simulink model "Collision_05_Disk_in_Ring"  (R2014a)
settings: Solver=ode15s  StartTime=0.0  StopTime=5  MaxStep=1e-2  RelTol=1e-4  AbsTol=1e-5
PostLoadFcn:
  | warning off Simulink:Engine:UsingDefaultMaxStepSize
StartFcn:
  | tic;
StopFcn:
  | Elapsed_Sim_Time = toc;
  | disp(['Elapsed Sim Time = ' num2str(Elapsed_Sim_Time)]);
undefined symbols (not defined in the file): X, Y, Z
libraries: sm_lib x6, Parts_Lib x2, nesl_utility x2, Contact_Forces_Lib x1
Description:
  | Copyright 2014 The MathWorks, Inc.
settings Model: Creator=smiller  LastModifiedBy=smiller
settings SolverCC: ZeroCrossAlgorithm=Adaptive
settings DataIOCC: LimitDataPoints=off
settings OptimizationCC: ExpressionDepthLimit=2147483647
settings DebuggingCC: UnderspecifiedInitializationDetection=Classic  IgnoredZcDiagnostic=none  FcnCallInpInsideContextMsg=EnableAllAsWarning  StateNameClashWarn=warning
settings DiagnosticsConfigSet: SimMechanicsRigidlyBoundBlock=none
settings ExplorerConfigSet: InternalSimMechanicsExplorerSettings="<ExplorerConfiguration><canonicalview>default</canonicalview><AnimationSetting><BasePlaybackSpeed>1.0</BasePlaybackSpeed><PlaybackSpeedFactor>1.0</PlaybackSpeedFactor></AnimationSetting><TilePanel><TileInfo><Tiles Columns=\"1\" Count=\"1\" Rows=\"1\"><Column Left=\"2\" Weight=\"1\"/><Column Left=\"392\"/><Row Top=\"2\" Weight=\"1\"/><Row Top=\"346\"/><Tile Height=\"1\" Width=\"1\" X=\"0\" Y=\"0\"/></Tiles></TileInfo><SceneInfo><SceneViewer><BGColor><R>0.92549020051956177</R><G>0.94901961088180542</G><B>0.94901961088180542</B></BGColor><Camera><Position><X>0.30265771427387711</X><Y>-0.55071230602769961</Y><Z>0.10379549062534259</Z></Position><Center><X>0.0025347841246010638</X><Y>0.0091500402941713244</Y><Z>0.0013498174437712174</Z></Center><Up><X>-0.17021912957199431</X><Y>0.088338633384022841</Y><Z>0.98143860418244988</Z></Up><Left>-0.23099999874830246</Left><Right>0.23099999874830246</Right><Bottom>-0.23099999874830246</Bottom><Top>0.23099999874830246</Top></Camera></SceneViewer></SceneInfo></TilePanel></ExplorerConfiguration>"

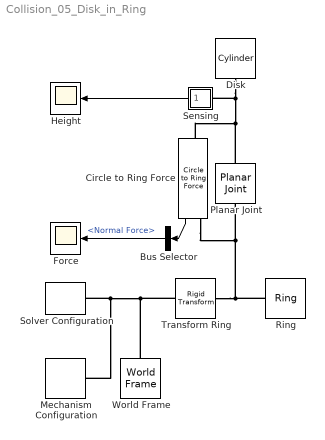
== system Collision_05_Disk_in_Ring ==
  Bus Selector : BusSelector  OutputSignals=Normal Force
  Circle to Ring Force : Contact_Forces_Lib/2D/Circle to Ring Force  radius_circle=0.05  radius_ring=0.21  d_ring=0.02  active_angle=[-180 180]  force_law=Linear  k_contact=1e4  b_contact=1e1  pen_full_damp_F=1e-4  pen_exponent=1  custom_param_1=1  custom_param_2=1  friction_law=None  mu_kinetic=0.5  mu_static=0.7  v_thr=0.001
  Disk : Parts_Lib/Cylinder  cyl_radius=0.05  cyl_length=0.05  cyl_density=1000  cyl_color=red  mark_radius=[0.75 0.5]  mark_angle=60  mark_color=purple
  Force : Scope
      settings: TimeRange=5  YMin=0  YMax=150
  Height : Scope
      settings: YMin=-0.2  YMax=0.2
  Mechanism Configuration : sm_lib/Utilities/Mechanism Configuration  UniformGravity=Constant  GravityVector=[0 0 -9.81]  GravityUnits=m/s^2  LinearizationDelta=0.001  BlockFunction=simmechanics.library.utilities.mechanism_configuration
  Planar Joint : sm_lib/Joints/Planar Joint  SenseConstraintForce=off  SenseConstraintForceX=off  SenseConstraintForceY=off  SenseConstraintForceZ=off  SenseConstraintTorque=off  SenseConstraintTorqueX=off  SenseConstraintTorqueY=off  SenseConstraintTorqueZ=off  SenseTotalForce=off  SenseTotalForceX=off  SenseTotalForceY=off  SenseTotalForceZ=off  SenseTotalTorque=off  SenseTotalTorqueX=off  SenseTotalTorqueY=off  SenseTotalTorqueZ=off  CompositeWrenchDir=FollowerOnBase  CompositeWrenchFrame=BaseFrame  PxEquilibriumPosition=0  PxEquilibriumPositionUnits=m  PxSpringStiffness=0  PxSpringStiffnessUnits=N/m  PxDampingCoefficient=0  PxDampingCoefficientUnits=N/(m/s)  PxTorqueActuationMode=NoTorque  PxMotionActuationMode=ComputedMotion  PxSensePosition=off  PxSenseVelocity=off  PxSenseAcceleration=off  PxSenseTorqueForce=off  PxPositionTargetValue=0.07  PxPositionTargetValueUnits=m  PxPositionTargetSpecify=on  PxPositionTargetPriority=High  PxVelocityTargetValue=0  PxVelocityTargetValueUnits=m/s  PxVelocityTargetSpecify=off  PxVelocityTargetPriority=High  PyEquilibriumPosition=0  PyEquilibriumPositionUnits=m  PySpringStiffness=0  PySpringStiffnessUnits=N/m  PyDampingCoefficient=0  PyDampingCoefficientUnits=N/(m/s)  PyTorqueActuationMode=NoTorque  PyMotionActuationMode=ComputedMotion  PySensePosition=off  PySenseVelocity=off  PySenseAcceleration=off  PySenseTorqueForce=off  PyPositionTargetValue=0.05  PyPositionTargetValueUnits=m  PyPositionTargetSpecify=on  PyPositionTargetPriority=High  PyVelocityTargetValue=0.5*0  PyVelocityTargetValueUnits=m/s  PyVelocityTargetSpecify=on  PyVelocityTargetPriority=High  RzEquilibriumPosition=0  RzEquilibriumPositionUnits=deg  RzSpringStiffness=0  RzSpringStiffnessUnits=N*m/deg  RzDampingCoefficient=0  RzDampingCoefficientUnits=N*m/(deg/s)  RzTorqueActuationMode=NoTorque  RzMotionActuationMode=ComputedMotion  RzSensePosition=off  RzSenseVelocity=off  RzSenseAcceleration=off  RzSenseTorqueForce=off  RzPositionTargetValue=0  RzPositionTargetValueUnits=deg  RzPositionTargetSpecify=off  RzPositionTargetPriority=High  RzVelocityTargetValue=0  RzVelocityTargetValueUnits=deg/s  RzVelocityTargetSpecify=off  RzVelocityTargetPriority=High  BlockFunction=simmechanics.library.joints.planar_joint
  Ring : Parts_Lib/Ring  outer_rad=0.22  inner_rad=0.2  ring_length=0.05  ring_density=1000  ring_color=gray  mark_radius=[0.98 1.02]  mark_angle=60  mark_color=black
  Sensing : Subsystem
      mask Display: disp('S')
  Solver Configuration : nesl_utility/Solver Configuration  PhysicalDomain=network_engine_domain  SubClassName=solver  LeftPortType=input  RightPortType=generic  Accelerate=off  Tones=[]  Harmonics=[]  SimulateNoise=off  Profile=off  UseLocalSampling=off  EnableSwitchedLinearOptims=on  FrequencyDomain=off  UseCCode=off  RelTol=0.001  AbsTol=1e-06  MinStep=1e-09  ToWorkspace=off  DoDC=off  ResidualTolerance=1e-9  UseLocalSolver=off  LocalSolverChoice=NE_BACKWARD_EULER_ADVANCER  LocalSolverSampleTime=.001  DoFixedCost=off  MaxNonlinIter=3  MaxModeIter=2  LinearAlgebra=Sparse  DelaysMemoryBudget=1024  AutomaticFiltering=on  FilteringTimeConstant=0.001
  Transform Ring : sm_lib/Frames and Transforms/Rigid Transform  TranslationMethod=None  TranslationLengthUnit=m  TranslationStandardAxis=+Z  TranslationStandardOffset=0  TranslationCartesianOffset=[0 0 0]  TranslationROffset=0  TranslationROffsetUnits=m  TranslationZOffset=0  TranslationZOffsetUnits=m  TranslationThetaOffset=0  TranslationThetaOffsetUnits=deg  RotationMethod=StandardAxis  RotationAngleUnits=deg  RotationStandardAxis=+X  RotationAngle=90  RotationArbitraryAxis=[0 0 1]  FollAlignAxisA=+X  BaseAlignAxisA=+Z  FollAlignAxisB=+Y  BaseAlignAxisB=+X  BlockFunction=simmechanics.library.frames_transforms.rigid_transform
  World Frame : sm_lib/Frames and Transforms/World Frame  BlockFunction=simmechanics.library.frames_transforms.world_frame
  wires:
  Sensing/1(S) -> Height/1
  Circle to Ring Force/1 -> Bus Selector/1
  Bus Selector/1 -> Force/1  "<Normal Force>"
  connections:
  Sensing/LConn1 -- Planar Joint/RConn1 -- Circle to Ring Force/LConn1 -- Disk/LConn1
  Circle to Ring Force/RConn1 -- Ring/LConn1 -- Transform Ring/RConn1 -- Planar Joint/LConn1
  Mechanism Configuration/RConn1 -- Transform Ring/LConn1 -- World Frame/RConn1 -- Solver Configuration/RConn1

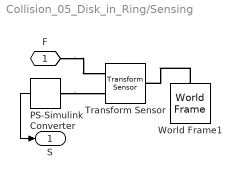
== system Collision_05_Disk_in_Ring/Sensing ==
  PS-Simulink Converter : nesl_utility/PS-Simulink Converter  PhysicalDomain=network_engine_domain  SubClassName=ps_output  LeftPortType=input  RightPortType=output  PseudoPeriodic=off  Frequencies=[]  Unit=1  AffineConversion=off
  Transform Sensor : sm_lib/Frames and Transforms/Transform Sensor  MeasurementFrame=World  SenseAngle=off  SenseAxis=off  SenseAngle1=off  SenseAngle2=off  SenseAngle3=off  SenseQ=off  SenseR=off  SenseOmegaX=off  SenseOmegaY=off  SenseOmegaZ=off  SenseOmega1=off  SenseOmega2=off  SenseOmega3=off  SenseQDot=off  SenseRDot=off  SenseAlphaX=off  SenseAlphaY=off  SenseAlphaZ=off  SenseAlpha1=off  SenseAlpha2=off  SenseAlpha3=off  SenseQDDot=off  SenseRDDot=off  SenseX=off  SenseY=off  SenseZ=on  SenseRad=off  SenseAzim=off  SenseDist=off  SenseInc=off  SenseXDot=off  SenseYDot=off  SenseZDot=off  SenseRadDot=off  SenseAzimDot=off  SenseDistDot=off  SenseIncDot=off  SenseXDDot=off  SenseYDDot=off  SenseZDDot=off  SenseRadDDot=off  SenseAzimDDot=off  SenseDistDDot=off  SenseIncDDot=off  BlockFunction=simmechanics.library.frames_transforms.transform_sensor
  World Frame1 : sm_lib/Frames and Transforms/World Frame  BlockFunction=simmechanics.library.frames_transforms.world_frame
  F : PMIOPort  Port=1  Side=Left
  S : Outport
  wires:
  PS-Simulink Converter/1 -> S/1
  connections:
  World Frame1/RConn1 -- Transform Sensor/LConn1
  F/RConn1 -- Transform Sensor/RConn1
  PS-Simulink Converter/LConn1 -- Transform Sensor/RConn2
